simulink model "SIR_Model"  (R2024b)
settings: Solver=FixedStepDiscrete  StartTime=0.0  StopTime=150  FixedStep=1  RelTol=1e-3
values from neighbouring files (symbols this model uses):
  a = 1/3    (= 0.333333333333)    [run_sir_model.m]
  b = 1.3    [run_sir_model.m]
  i0 = I0/N    (= 1.26582278481e-06)    [run_sir_model.m]
  r0 = R0/N    (= 0)    [run_sir_model.m]
  s0 = S0/N    (= 0.999998734177)    [run_sir_model.m]

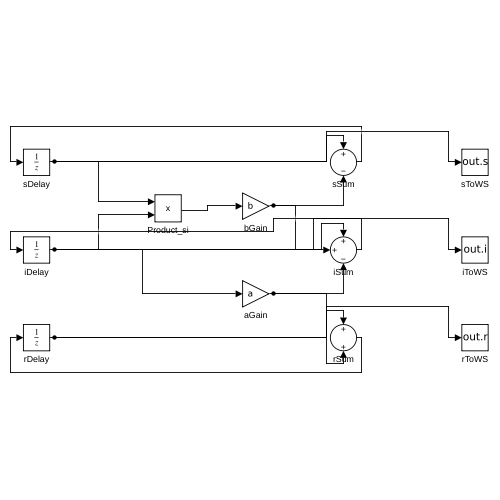
[thumbnail: Simulink's stored preview of the top-level diagram]
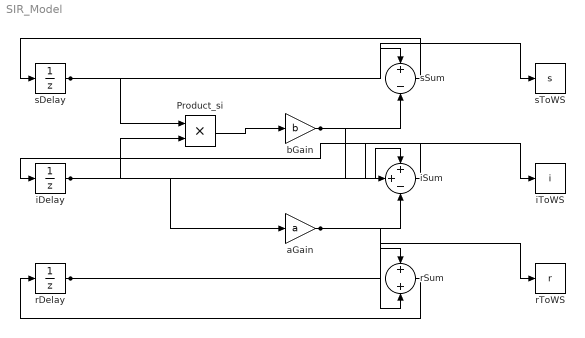
== system SIR_Model ==
  Product_si : Product
  aGain : Gain  Gain=a
  bGain : Gain  Gain=b
  iDelay : UnitDelay  InitialCondition=i0  SampleTime=-1  HasFrameUpgradeWarning=on
  iSum : Sum  Inputs=++-
  iToWS : ToWorkspace  VariableName=i  SaveFormat=Structure With Time  SampleTime=-1
  rDelay : UnitDelay  InitialCondition=r0  SampleTime=-1  HasFrameUpgradeWarning=on
  rSum : Sum
  rToWS : ToWorkspace  VariableName=r  SaveFormat=Structure With Time  SampleTime=-1
  sDelay : UnitDelay  InitialCondition=s0  SampleTime=-1  HasFrameUpgradeWarning=on
  sSum : Sum  Inputs=+-
  sToWS : ToWorkspace  VariableName=s  SaveFormat=Structure With Time  SampleTime=-1
  wires:
  sDelay/1 -> sSum/1, Product_si/1, sToWS/1
  iDelay/1 -> iSum/1, Product_si/2, aGain/1, iToWS/1
  Product_si/1 -> bGain/1
  bGain/1 -> sSum/2, iSum/2
  aGain/1 -> iSum/3, rSum/2
  rDelay/1 -> rSum/1, rToWS/1
  sSum/1 -> sDelay/1
  iSum/1 -> iDelay/1
  rSum/1 -> rDelay/1
